simulink model "test_clump_resync_unclump"  (Simulink 7.4)
settings: Solver=ode45  StartTime=0  StopTime=500  RelTol=1e-3
libraries: xbsIndex_r4 x60, isi_correlator_lib x3, xps_library x1
settings Model: Creator=wjm  LastModifiedBy=wjm

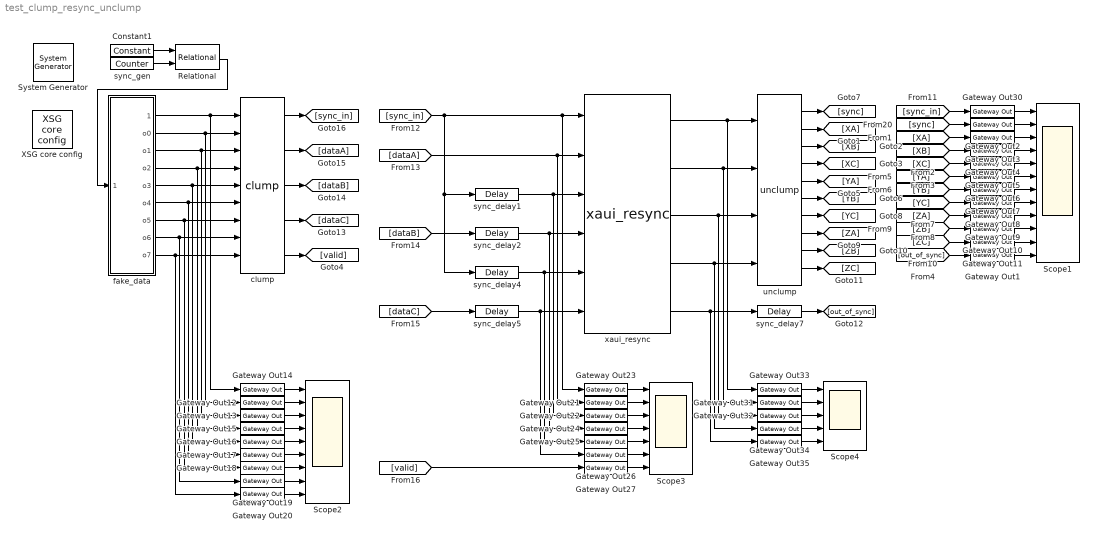
== system test_clump_resync_unclump ==
  " System Generator" : xbsIndex_r4/ System Generator  Tag=genX  SystemSampleTime=-1  xilinxfamily=virtex5  part=xc5vsx95t  speed=-1  package=ff1136  synthesis_tool=XST  clock_wrapper=Clock Enables  directory=./test_link_mux_demux/sysgen  testbench=off  simulink_period=1  sysclk_period=5  dcm_input_clock_period=100  incr_netlist=off  trim_vbits=Everywhere in SubSystem  dbl_ovrd=According to Block Masks  core_generation=According to Block Masks  run_coregen=off  deprecated_control=off  eval_field=0  block_type=sysgen
      settings: block_version=10.1.1
  Constant1 : xbsIndex_r4/Constant  arith_type=Unsigned  const=15  n_bits=7  bin_pt=0  explicit_period=on  period=1  equ=P=C  opselect=C  inp2=PCIN>>17  opr=+  inp1=P  carry=CIN  dbl_ovrd=off  block_type=constant
  Gateway Out{1..27,30..35} (33 alike) : xbsIndex_r4/Gateway Out  hdl_port=on  timing_constraint=None  locs_specified=off  LOCs={}  block_type=gatewayout
      settings: infoedit="Gateway out block.  Converts Xilinx fixed point inputs into ouputs of type Simulink integer, double, or fixed point.<br><br>Hardware notes:  In hardware these blocks become top level output ports or are discarded, depending on how they are configured."  block_version=11.3
  Relational : xbsIndex_r4/Relational  mode=a=b  en=off  latency=1  dbl_ovrd=off  block_type=relational
  Scope1 : Scope  NumInputPorts=12
      settings: YMin=-5~-5~-5~-5~-5~-5~-5~-5~-5~-5~-5~-5  YMax=5~5~5~5~5~5~5~5~5~5~5~5
  Scope2 : Scope  NumInputPorts=9
      settings: YMin=-5~-5~-5~-5~-5~-5~-5~-5~-5  YMax=5~5~5~5~5~5~5~5~5  SaveName=ScopeData4
  Scope3 : Scope  NumInputPorts=7
      settings: YMin=-5~-5~-5~-5~-5~-5~-5  YMax=5~5~5~5~5~5~5  SaveName=ScopeData5
  Scope4 : Scope  NumInputPorts=5
      settings: YMin=-5~-5~-5~-5~-5  YMax=5~5~5~5~5
  XSG core config : xps_library/XSG core config  Tag=xps:xsg  SystemSampleTime=-1  hw_sys=ROACH:sx95t  ibob_linux=off  clk_src=sys_clk2x  iBOB_clk_src=sys_clk  BEE2_ctrl_clk_src=sys_clk  BEE2_usr_clk_src=sys_clk  ROACH_clk_src=sys_clk2x  CORR_clk_src=sys_clk  gpio_clk_io_group=iBOB:sma  gpio_clk_bit_index=0  clk_rate=200  sample_period=1  synthesis_tool=XST  mpc_type=powerpc440_ext
  clump : isi_correlator_lib/clump  SystemSampleTime=-1  latency=1
  fake_data : Subsystem
  sync_delay1 : xbsIndex_r4/Delay  en=off  latency=11  dbl_ovrd=off  reg_retiming=off  block_type=delay
  sync_delay2 : xbsIndex_r4/Delay  en=off  latency=11  dbl_ovrd=off  reg_retiming=off  block_type=delay
  sync_delay4 : xbsIndex_r4/Delay  en=off  latency=17  dbl_ovrd=off  reg_retiming=off  block_type=delay
  sync_delay5 : xbsIndex_r4/Delay  en=off  latency=17  dbl_ovrd=off  reg_retiming=off  block_type=delay
  sync_delay7 : xbsIndex_r4/Delay  en=off  latency=1  dbl_ovrd=off  reg_retiming=off  block_type=delay
  sync_gen : xbsIndex_r4/Counter  cnt_type=Free Running  cnt_to=Inf  operation=Up  start_count=0  cnt_by_val=1  arith_type=Unsigned  n_bits=7  bin_pt=0  load_pin=off  rst=off  en=off  explicit_period=on  period=1  dbl_ovrd=off  use_behavioral_HDL=off  implementation=Fabric  use_rpm=off  block_type=counter
  unclump : isi_correlator_lib/unclump  SystemSampleTime=-1  latency=1
  xaui_resync : isi_correlator_lib/xaui_resync  SystemSampleTime=-1  buffer_depth=5  logic_latency=1
  wires:
  unclump/2 -> [XA]
  unclump/3 -> [XB]
  unclump/4 -> [XC]
  unclump/5 -> [YA]
  unclump/6 -> [YB]
  unclump/7 -> [YC]
  unclump/8 -> [ZA]
  unclump/9 -> [ZB]
  unclump/10 -> [ZC]
  fake_data/2(o0) -> clump/2, Gateway Out12/1
  fake_data/3(o1) -> clump/3, Gateway Out13/1
  fake_data/4(o2) -> clump/4, Gateway Out15/1
  fake_data/5(o3) -> clump/5, Gateway Out16/1
  fake_data/6(o4) -> clump/6, Gateway Out17/1
  fake_data/7(o5) -> clump/7, Gateway Out18/1
  fake_data/8(o6) -> clump/8, Gateway Out19/1
  fake_data/9(o7) -> clump/9, Gateway Out20/1
  Gateway Out14/1 -> Scope2/1
  Gateway Out12/1 -> Scope2/2
  Gateway Out13/1 -> Scope2/3
  Gateway Out15/1 -> Scope2/4
  Gateway Out16/1 -> Scope2/5
  Gateway Out17/1 -> Scope2/6
  Gateway Out18/1 -> Scope2/7
  Gateway Out19/1 -> Scope2/8
  Gateway Out20/1 -> Scope2/9
  fake_data/1(sync_out) -> clump/1, Gateway Out14/1
  [XA] -> Gateway Out3/1
  [XB] -> Gateway Out4/1
  [XC] -> Gateway Out5/1
  [YA] -> Gateway Out6/1
  [YB] -> Gateway Out7/1
  [YC] -> Gateway Out8/1
  [ZA] -> Gateway Out9/1
  [ZB] -> Gateway Out10/1
  unclump/1 -> [sync]
  [ZC] -> Gateway Out11/1
  [sync] -> Gateway Out2/1
  clump/1 -> [sync_in]
  clump/2 -> [dataA]
  clump/3 -> [dataB]
  clump/4 -> [dataC]
  clump/5 -> [valid]
  [sync_in] -> Gateway Out23/1, xaui_resync/1, sync_delay4/1, sync_delay1/1
  [dataA] -> Gateway Out21/1, xaui_resync/2
  [dataB] -> sync_delay2/1
  [dataC] -> sync_delay5/1
  sync_delay2/1 -> Gateway Out24/1, xaui_resync/4
  sync_delay1/1 -> Gateway Out22/1, xaui_resync/3
  sync_delay5/1 -> Gateway Out26/1, xaui_resync/6
  sync_delay4/1 -> Gateway Out25/1, xaui_resync/5
  xaui_resync/5 -> sync_delay7/1, Gateway Out35/1
  Gateway Out23/1 -> Scope3/1
  Gateway Out21/1 -> Scope3/2
  Gateway Out22/1 -> Scope3/3
  Gateway Out24/1 -> Scope3/4
  Gateway Out25/1 -> Scope3/5
  Gateway Out26/1 -> Scope3/6
  Gateway Out27/1 -> Scope3/7
  xaui_resync/1 -> Gateway Out33/1, unclump/1
  xaui_resync/2 -> Gateway Out31/1, unclump/2
  xaui_resync/3 -> Gateway Out32/1, unclump/3
  xaui_resync/4 -> Gateway Out34/1, unclump/4
  sync_delay7/1 -> [out_of_sync]
  [out_of_sync] -> Gateway Out1/1
  [sync_in] -> Gateway Out30/1
  Gateway Out30/1 -> Scope1/1
  Gateway Out2/1 -> Scope1/2
  Gateway Out3/1 -> Scope1/3
  Gateway Out4/1 -> Scope1/4
  Gateway Out5/1 -> Scope1/5
  Gateway Out6/1 -> Scope1/6
  Gateway Out7/1 -> Scope1/7
  Gateway Out8/1 -> Scope1/8
  Gateway Out9/1 -> Scope1/9
  Gateway Out10/1 -> Scope1/10
  Gateway Out11/1 -> Scope1/11
  Gateway Out1/1 -> Scope1/12
  Gateway Out33/1 -> Scope4/1
  Gateway Out31/1 -> Scope4/2
  Gateway Out32/1 -> Scope4/3
  Gateway Out34/1 -> Scope4/4
  Gateway Out35/1 -> Scope4/5
  Constant1/1 -> Relational/1
  sync_gen/1 -> Relational/2
  Relational/1 -> fake_data/1(sync)
  [valid] -> Gateway Out27/1

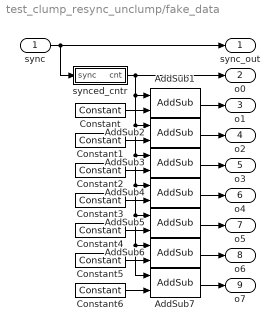
== system test_clump_resync_unclump/fake_data ==
  sync : Inport
  AddSub{1..7} (7 alike) : xbsIndex_r4/AddSub  mode=Addition  use_carryin=off  use_carryout=off  en=off  latency=0  precision=User Defined  arith_type=Unsigned  n_bits=8  bin_pt=0  quantization=Truncate  overflow=Wrap  dbl_ovrd=off  use_behavioral_HDL=off  hw_selection=Fabric  pipelined=off  block_type=addsub
  Constant : xbsIndex_r4/Constant  arith_type=Unsigned  const=1  n_bits=3  bin_pt=0  explicit_period=on  period=1  equ=P=C  opselect=C  inp2=PCIN>>17  opr=+  inp1=P  carry=CIN  dbl_ovrd=off  block_type=constant
      settings: block_version=11.4
  Constant1 : xbsIndex_r4/Constant  arith_type=Unsigned  const=2  n_bits=3  bin_pt=0  explicit_period=on  period=1  equ=P=C  opselect=C  inp2=PCIN>>17  opr=+  inp1=P  carry=CIN  dbl_ovrd=off  block_type=constant
      settings: block_version=11.4
  Constant2 : xbsIndex_r4/Constant  arith_type=Unsigned  const=3  n_bits=3  bin_pt=0  explicit_period=on  period=1  equ=P=C  opselect=C  inp2=PCIN>>17  opr=+  inp1=P  carry=CIN  dbl_ovrd=off  block_type=constant
      settings: block_version=11.4
  Constant3 : xbsIndex_r4/Constant  arith_type=Unsigned  const=4  n_bits=3  bin_pt=0  explicit_period=on  period=1  equ=P=C  opselect=C  inp2=PCIN>>17  opr=+  inp1=P  carry=CIN  dbl_ovrd=off  block_type=constant
      settings: block_version=11.4
  Constant4 : xbsIndex_r4/Constant  arith_type=Unsigned  const=5  n_bits=3  bin_pt=0  explicit_period=on  period=1  equ=P=C  opselect=C  inp2=PCIN>>17  opr=+  inp1=P  carry=CIN  dbl_ovrd=off  block_type=constant
      settings: block_version=11.4
  Constant5 : xbsIndex_r4/Constant  arith_type=Unsigned  const=6  n_bits=3  bin_pt=0  explicit_period=on  period=1  equ=P=C  opselect=C  inp2=PCIN>>17  opr=+  inp1=P  carry=CIN  dbl_ovrd=off  block_type=constant
      settings: block_version=11.4
  Constant6 : xbsIndex_r4/Constant  arith_type=Unsigned  const=7  n_bits=3  bin_pt=0  explicit_period=on  period=1  equ=P=C  opselect=C  inp2=PCIN>>17  opr=+  inp1=P  carry=CIN  dbl_ovrd=off  block_type=constant
      settings: block_version=11.4
  synced_cntr : Subsystem  AncestorBlock=isi_correlator_lib/synced_cntr  mask(synced_cntr){bitwidth=8}
      mask prompts: bitwidth "Counter bitwidth:"
      mask help: A counter that realigns itself with sync pulses.
  sync_out : Outport
  o0 : Outport  Port=2
  o1 : Outport  Port=3
  o2 : Outport  Port=4
  o3 : Outport  Port=5
  o4 : Outport  Port=6
  o5 : Outport  Port=7
  o6 : Outport  Port=8
  o7 : Outport  Port=9
  wires:
  Constant/1 -> AddSub1/2
  Constant1/1 -> AddSub2/2
  Constant2/1 -> AddSub3/2
  Constant3/1 -> AddSub4/2
  Constant4/1 -> AddSub5/2
  Constant5/1 -> AddSub6/2
  Constant6/1 -> AddSub7/2
  AddSub2/1 -> o2/1
  AddSub3/1 -> o3/1
  AddSub4/1 -> o4/1
  AddSub5/1 -> o5/1
  AddSub6/1 -> o6/1
  AddSub7/1 -> o7/1
  synced_cntr/1(cnt) -> AddSub1/1, AddSub2/1, AddSub3/1, AddSub4/1, AddSub5/1, AddSub7/1, AddSub6/1, o0/1
  sync/1 -> sync_out/1, synced_cntr/1(sync)
  AddSub1/1 -> o1/1

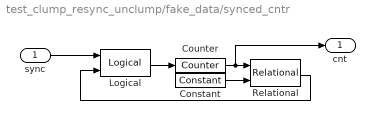
== system test_clump_resync_unclump/fake_data/synced_cntr ==
  sync : Inport
  Constant : xbsIndex_r4/Constant  arith_type=Unsigned  const=2^bitwidth - 2  n_bits=bitwidth  bin_pt=0  explicit_period=on  period=1  equ=P=C  opselect=C  inp2=PCIN>>17  opr=+  inp1=P  carry=CIN  dbl_ovrd=off  block_type=constant
      settings: block_version=10.1.1
  Counter : xbsIndex_r4/Counter  cnt_type=Free Running  cnt_to=Inf  operation=Up  start_count=0  cnt_by_val=8  arith_type=Unsigned  n_bits=bitwidth  bin_pt=0  load_pin=off  rst=on  en=off  explicit_period=on  period=1  dbl_ovrd=off  use_behavioral_HDL=off  implementation=Fabric  use_rpm=off  block_type=counter
  Logical : xbsIndex_r4/Logical  logical_function=AND  inputs=2  en=off  latency=0  precision=Full  arith_type=Unsigned  n_bits=16  bin_pt=0  align_bp=on  dbl_ovrd=off  block_type=logical
      settings: block_version=11.3
  Relational : xbsIndex_r4/Relational  mode=a!=b  en=off  latency=1  dbl_ovrd=off  block_type=relational
  cnt : Outport
  wires:
  Logical/1 -> Counter/1
  Counter/1 -> cnt/1, Relational/1
  Constant/1 -> Relational/2
  Relational/1 -> Logical/2
  sync/1 -> Logical/1
